simulink model "simul12"  (R2016b)
settings: Solver=ode4  StartTime=0.0  StopTime=1  FixedStep=0.001  RelTol=1e-3
values from neighbouring files (symbols this model uses):
  Ka = 4.5    [Problema12.m]
  Kdc = 1.1    [Problema12.m]
  Ki = 14.3    [Problema12.m]
  Kr = -0.37    [Problema12.m]
  w_a = 150    [Problema12.m]
  z_a = 0.7    [Problema12.m]
settings Model: Creator=David  LastModifiedBy=josed

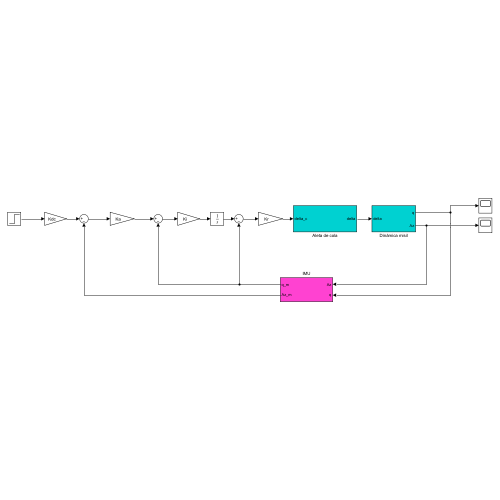
[thumbnail: Simulink's stored preview of the top-level diagram]
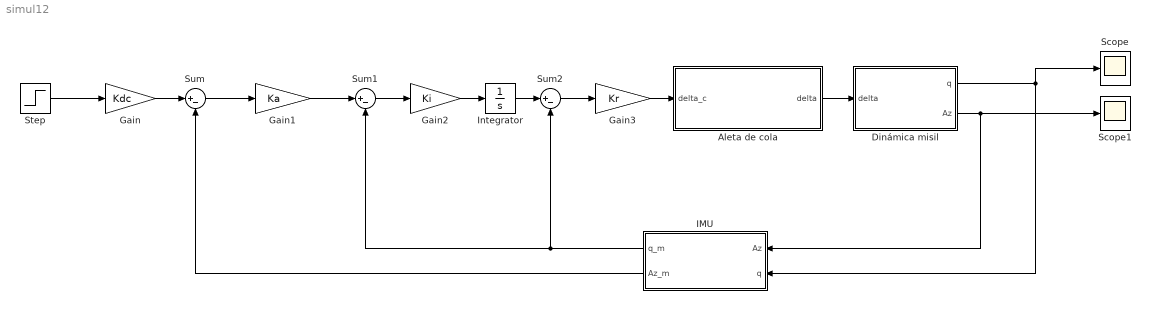
== system simul12 ==
  Aleta de cola : Subsystem
  Dinámica misil : Subsystem
  Gain : Gain  Gain=Kdc
  Gain1 : Gain  Gain=Ka
  Gain2 : Gain  Gain=Ki
  Gain3 : Gain  Gain=Kr
  IMU : Subsystem
  Integrator : Integrator
  Scope : Scope
  Scope1 : Scope
  Step : Step  Time=0  SampleTime=0
  Sum : Sum  Inputs=|+-
  Sum1 : Sum  Inputs=|+-
  Sum2 : Sum  Inputs=|+-
  wires:
  Step/1 -> Gain/1
  Gain/1 -> Sum/1
  Sum/1 -> Gain1/1
  Gain1/1 -> Sum1/1
  Sum1/1 -> Gain2/1
  Gain2/1 -> Integrator/1
  Integrator/1 -> Sum2/1
  Sum2/1 -> Gain3/1
  Gain3/1 -> Aleta de cola/1(delta_c)
  Aleta de cola/1(delta) -> Dinámica misil/1(delta)
  Dinámica misil/2(Az) -> IMU/1(Az), Scope1/1
  Dinámica misil/1(q) -> IMU/2(q), Scope/1
  IMU/1(q_m) -> Sum1/2, Sum2/2
  IMU/2(Az_m) -> Sum/2

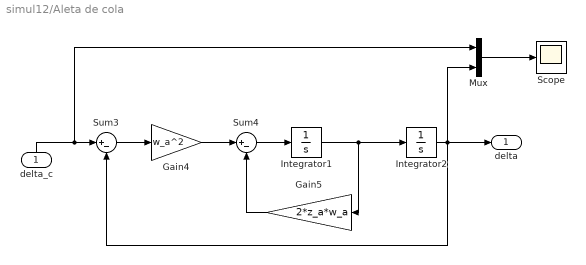
== system simul12/Aleta de cola ==
  delta_c : Inport
  Gain4 : Gain  Gain=w_a^2
  Gain5 : Gain  Gain=2*z_a*w_a
  Integrator1 : Integrator
  Integrator2 : Integrator
  Mux : Mux  Inputs=2
  Scope : Scope
  Sum3 : Sum  Inputs=|+-
  Sum4 : Sum  Inputs=|+-
  delta : Outport
  wires:
  Sum4/1 -> Integrator1/1
  delta_c/1 -> Mux/1, Sum3/1
  Gain5/1 -> Sum4/2
  Integrator1/1 -> Gain5/1, Integrator2/1
  Integrator2/1 -> Mux/2, delta/1, Sum3/2
  Gain4/1 -> Sum4/1
  Sum3/1 -> Gain4/1
  Mux/1 -> Scope/1

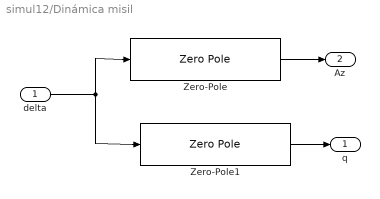
== system simul12/Dinámica misil ==
  delta : Inport
  Zero-Pole : ZeroPole  Zeros=[-34.3 34.3]  Poles=[-0.56-9.32j -0.56+9.32j]  Gain=[0.2038]
  Zero-Pole1 : ZeroPole  Zeros=[-1]  Poles=[-0.56-9.32j -0.56+9.32j]  Gain=[-131]
  q : Outport
  Az : Outport  Port=2
  wires:
  Zero-Pole/1 -> Az/1
  delta/1 -> Zero-Pole1/1, Zero-Pole/1
  Zero-Pole1/1 -> q/1

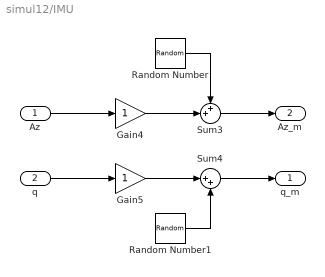
== system simul12/IMU ==
  Az : Inport
  q : Inport  Port=2
  Gain4 : Gain
  Gain5 : Gain
  Random Number : RandomNumber  Variance=1e-3  Seed=654321  SampleTime=0.001
  Random Number1 : RandomNumber  Variance=1e-4  Seed=654321  SampleTime=0.001
  Sum3 : Sum  Inputs=++|
  Sum4 : Sum  Inputs=|++
  q_m : Outport
  Az_m : Outport  Port=2
  wires:
  Sum4/1 -> q_m/1
  Random Number/1 -> Sum3/1
  Az/1 -> Gain4/1
  Sum3/1 -> Az_m/1
  q/1 -> Gain5/1
  Random Number1/1 -> Sum4/2
  Gain4/1 -> Sum3/2
  Gain5/1 -> Sum4/1
